simulink model "sim_near_pi"  (R2020b)
settings: Solver=ode45  StartTime=0.0  StopTime=10.0  MaxStep=0.5e-3  RelTol=1e-6
values from neighbouring files (symbols this model uses):
  s_star = C_features_desired(:)    [init.m]
libraries: simulink x1
settings Model: Creator=marco  LastModifiedBy=marco

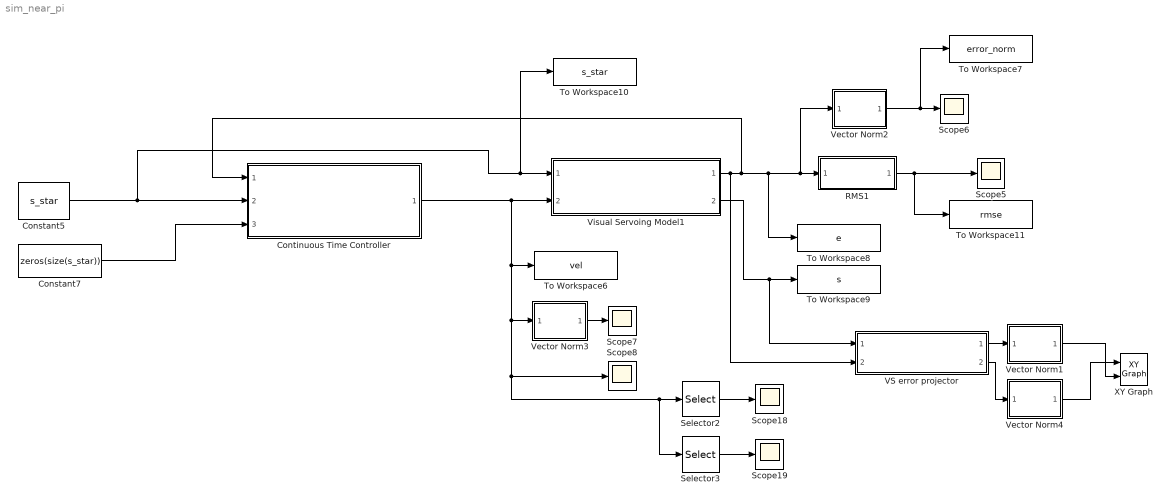
== system sim_near_pi ==
  Constant5 : Constant  Value=s_star
  Constant7 : Constant  Value=zeros(size(s_star))
  Continuous Time Controller : Subsystem  ReferencedSubsystem=continuous_time_controller  lambda=5  forward_action_enabled=off
  RMS1 : Subsystem  ReferencedSubsystem=RMS
  Scope{5..8,18..19} (6 alike) : Scope
  Selector2 : Selector  InputPortWidth=6  IndexOptions=Index vector (dialog)  Indices=1:3  OutputSizes=1
  Selector3 : Selector  InputPortWidth=6  IndexOptions=Index vector (dialog)  Indices=4:6  OutputSizes=1
  To Workspace10 : ToWorkspace  VariableName=s_star  SaveFormat=Timeseries  SampleTime=-1
  To Workspace11 : ToWorkspace  VariableName=rmse  SaveFormat=Timeseries  SampleTime=-1
  To Workspace6 : ToWorkspace  VariableName=vel  SaveFormat=Timeseries  SampleTime=-1
  To Workspace7 : ToWorkspace  VariableName=error_norm  SaveFormat=Timeseries  SampleTime=-1
  To Workspace8 : ToWorkspace  VariableName=e  SaveFormat=Timeseries  SampleTime=-1
  To Workspace9 : ToWorkspace  VariableName=s  SaveFormat=Timeseries  SampleTime=-1
  VS error projector : Subsystem  ReferencedSubsystem=LProj
  Vector Norm{1..4} (4 alike) : Subsystem  ReferencedSubsystem=Norm
  Visual Servoing Model1 : Subsystem  ReferencedSubsystem=Features_System  s0=s0  noise_perc=0  noise_sample_time=1
  XY Graph : simulink/Sinks/XY Graph  xmin=0  xmax=1  ymin=0  ymax=1  st=0.001
  wires:
  Constant7/1 -> Continuous Time Controller/3
  Visual Servoing Model1/2 -> VS error projector/1, To Workspace9/1
  Vector Norm3/1 -> Scope7/1
  Vector Norm2/1 -> Scope6/1, To Workspace7/1
  RMS1/1 -> Scope5/1, To Workspace11/1
  Visual Servoing Model1/1 -> VS error projector/2, Continuous Time Controller/1, RMS1/1, Vector Norm2/1, To Workspace8/1
  Constant5/1 -> Continuous Time Controller/2, Visual Servoing Model1/1, To Workspace10/1
  Selector2/1 -> Scope18/1
  Selector3/1 -> Scope19/1
  Continuous Time Controller/1 -> Visual Servoing Model1/2, Vector Norm3/1, Selector3/1, Selector2/1, Scope8/1, To Workspace6/1
  VS error projector/1 -> Vector Norm1/1
  VS error projector/2 -> Vector Norm4/1
  Vector Norm4/1 -> XY Graph/1
  Vector Norm1/1 -> XY Graph/2
